simulink model "SimulinkExamen"  (R2019a)
settings: Solver=VariableStepAuto  StartTime=0.0  StopTime=10.0  RelTol=1e-3
libraries: fuzblock x1
settings Model: Creator=user  LastModifiedBy=user

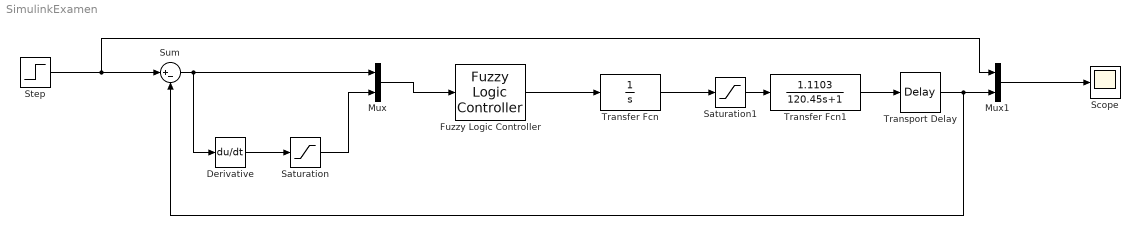
== system SimulinkExamen ==
  Derivative : Derivative
  Fuzzy Logic Controller : fuzblock/Fuzzy Logic  Controller  FIS='tipper.fis'  OutputSampleNumber=101  DataType=double  FuzzifiedInputs=off  RuleFiringStrengths=off  RuleOutputs=off  AggregatedOutputs=off  SimulateUsing=Interpreted execution  OutOfRangeInputValueMessage=warning  NoRuleFiredMessage=warning  EmptyOutputFuzzySetMessage=warning
  Mux : Mux  Inputs=2
  Mux1 : Mux  Inputs=2
  Saturation : Saturate
  Saturation1 : Saturate
  Scope : Scope
  Step : Step  SampleTime=0
  Sum : Sum  Inputs=|+-
  Transfer Fcn : TransferFcn  Denominator=[1 0]
  Transfer Fcn1 : TransferFcn  Numerator=[1.1103]  Denominator=[120.45 1]
  Transport Delay : TransportDelay
  wires:
  Transfer Fcn1/1 -> Transport Delay/1
  Saturation1/1 -> Transfer Fcn1/1
  Transfer Fcn/1 -> Saturation1/1
  Fuzzy Logic Controller/1 -> Transfer Fcn/1
  Mux1/1 -> Scope/1
  Mux/1 -> Fuzzy Logic Controller/1
  Saturation/1 -> Mux/2
  Derivative/1 -> Saturation/1
  Step/1 -> Mux1/1, Sum/1
  Sum/1 -> Mux/1, Derivative/1
  Transport Delay/1 -> Sum/2, Mux1/2
